simulink model "assignemnt_simulink"  (R2018b)
settings: Solver=FixedStepAuto  StartTime=0.0  StopTime=4  FixedStep=0.1  RelTol=1e-3
settings Model: Creator=mario  LastModifiedBy=jianhuili
settings SolverCC: ZeroCrossAlgorithm=Adaptive
settings DebuggingCC: IgnoredZcDiagnostic=none
settings SFSimCC: SimUseLocalCustomCode=off
settings RTWCC: RTWUseLocalCustomCode=off

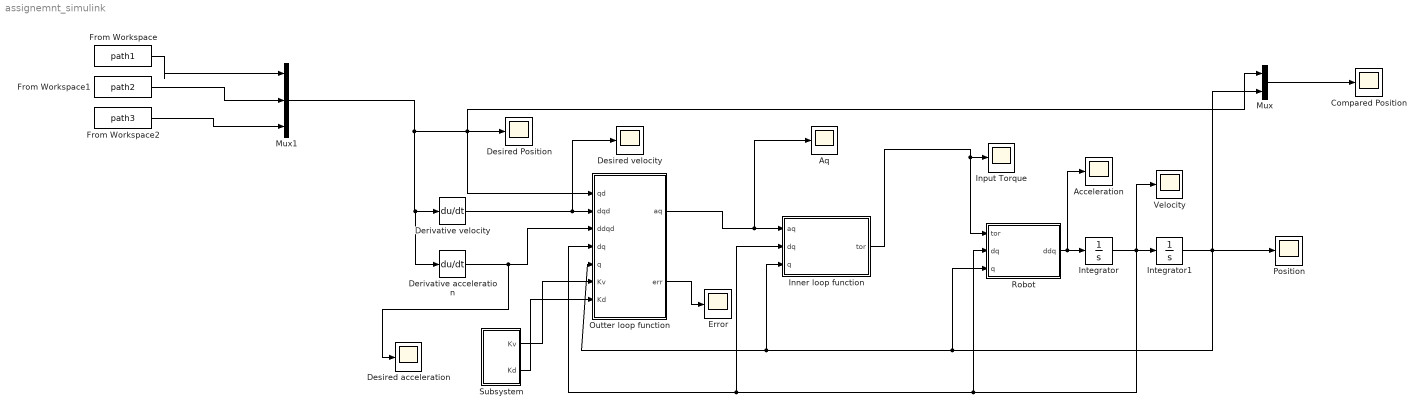
== system assignemnt_simulink ==
  Acceleration : Scope
  Aq : Scope
  Compared Position : Scope
  Derivative acceleration : Derivative  CoefficientInTFapproximation=0
  Derivative velocity : Derivative  CoefficientInTFapproximation=0
  Desired Position : Scope
  Desired acceleration : Scope
  "Desired velocity " : Scope
  Error : Scope
  From Workspace : FromWorkspace  VariableName=path1  SampleTime=0.1  Interpolate=off  OutputAfterFinalValue=Setting to zero
  From Workspace1 : FromWorkspace  VariableName=path2  SampleTime=0.1  Interpolate=off  OutputAfterFinalValue=Setting to zero
  From Workspace2 : FromWorkspace  VariableName=path3  SampleTime=0.1  Interpolate=off  OutputAfterFinalValue=Setting to zero
  Inner loop function : MATLAB Function  TreatAsAtomicUnit=on
  Input Torque : Scope
  Integrator : Integrator  InitialCondition=[0,0,0]
  Integrator1 : Integrator  InitialCondition=[0,0,0]
  Mux : Mux  Inputs=2
  Mux1 : Mux  Inputs=3
  Outter loop function : MATLAB Function  TreatAsAtomicUnit=on
  "Position " : Scope
  Robot : MATLAB Function  TreatAsAtomicUnit=on
  Subsystem : Subsystem
  Velocity : Scope
  wires:
  Outter loop function/2(err) -> Error/1
  Outter loop function/1(aq) -> Aq/1, Inner loop function/1(aq)
  Inner loop function/1(tor) -> Robot/1(tor), Input Torque/1
  Mux/1 -> Compared Position/1
  Robot/1(ddq) -> Acceleration/1, Integrator/1
  Integrator1/1 -> Mux/2, "Position "/1, Robot/3(q), Inner loop function/3(q), Outter loop function/5(q)
  Integrator/1 -> Robot/2(dq), Inner loop function/2(dq), Outter loop function/4(dq), Velocity/1, Integrator1/1
  Subsystem/1(Kv) -> Outter loop function/6(Kv)
  Subsystem/2(Kd) -> Outter loop function/7(Kd)
  Derivative velocity/1 -> "Desired velocity "/1, Outter loop function/2(dqd)
  Mux1/1 -> Mux/1, Outter loop function/1(qd), Desired Position/1, Derivative acceleration/1, Derivative velocity/1
  Derivative acceleration/1 -> Desired acceleration/1, Outter loop function/3(ddqd)
  From Workspace1/1 -> Mux1/2
  From Workspace2/1 -> Mux1/3
  From Workspace/1 -> Mux1/1

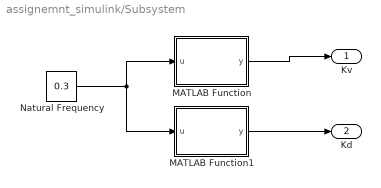
== system assignemnt_simulink/Subsystem ==
  MATLAB Function : MATLAB Function  TreatAsAtomicUnit=on
  MATLAB Function1 : MATLAB Function  TreatAsAtomicUnit=on
  Natural Frequency : Constant  Value=0.3
  Kv : Outport
  Kd : Outport  Port=2
  wires:
  Natural Frequency/1 -> MATLAB Function1/1(u), MATLAB Function/1(u)
  MATLAB Function1/1(y) -> Kd/1
  MATLAB Function/1(y) -> Kv/1

== matlab function assignemnt_simulink/Inner loop function ==
  data: aq input; dq input; q input; tor output
function tor = RPRlinkdyn(aq,dq,q)
coder.extrinsic('innerfunction');
tor = zeros(3,1);
tor=innerfunction(q,dq,aq);

end

== matlab function assignemnt_simulink/Outter loop function ==
  data: qd input; aq output; dqd input; ddqd input; dq input; q input; Kv input; Kd input; err output
function [aq,err] = control(qd,dqd,ddqd,dq,q,Kv,Kd)
% controls example for MSE 4401
 
aq = ddqd-Kd*(q-qd)-Kv*(dq-dqd);
err = [qd-q];

== matlab function assignemnt_simulink/Robot ==
  data: tor input; dq input; q input; ddq output
function ddq = RPRlinkdyn(tor,dq,q)
coder.extrinsic('robot');
ddq = zeros(3,1);
ddq=robot(q,dq,tor);
end

== matlab function assignemnt_simulink/Subsystem/MATLAB Function ==
  data: u input; y output
function y = dergain(u)

y = [2*u 0 0
    0 2*u 0
    0 0 2*u];

== matlab function assignemnt_simulink/Subsystem/MATLAB Function1 ==
  data: u input; y output
function y = postgain(u)

y = [u*u 0 0
    0 u*u 0
    0 0 u*u];
